simulink model "beam_mass_simulink_old"  (R2017a)
settings: Solver=FixedStepAuto  StartTime=0.0  StopTime=100  FixedStep=0.01  RelTol=1e-3
libraries: simulink_extras x2, simulink x1
settings Model: Creator=gladstonjoseph  LastModifiedBy=gladstonjoseph
settings DataIOCC: ReturnWorkspaceOutputs=on
settings DebuggingCC: UnconnectedInputMsg=none  UnconnectedOutputMsg=none  UnconnectedLineMsg=none
settings ModelReferenceCC: EnableRefExpFcnMdlSchedulingChecks=off
settings SFSimCC: SimUseLocalCustomCode=on
settings RTWCC: RTWUseLocalCustomCode=on

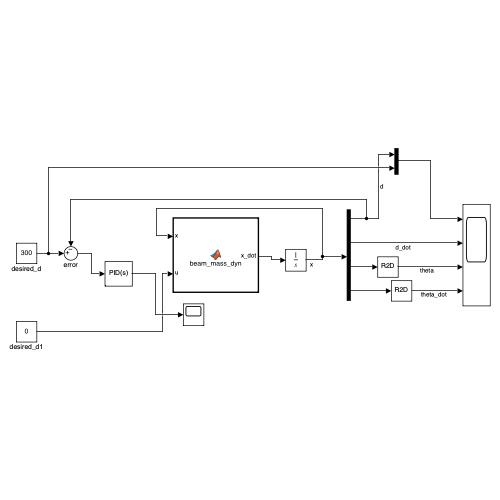
[thumbnail: Simulink's stored preview of the top-level diagram]
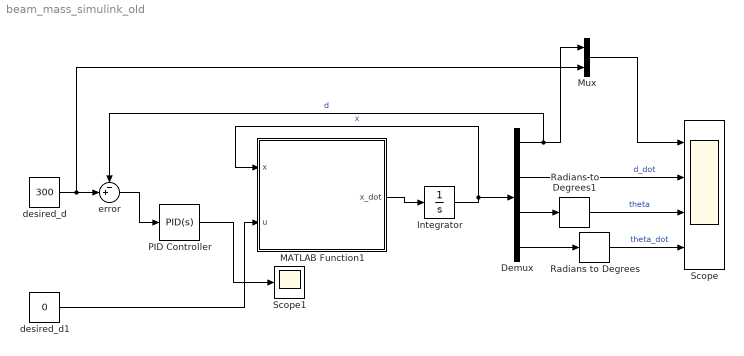
== system beam_mass_simulink_old ==
  Demux : Demux
  Integrator : Integrator  InitialCondition=[0, 0, 0.0001, 0]'
  MATLAB Function1 : MATLAB Function  TreatAsAtomicUnit=on
  Mux : Mux  Inputs=2
  PID Controller : simulink/Continuous/PID Controller  Controller=PID  Form=Parallel  TimeDomain=Continuous-time  SampleTime=-1  IntegratorMethod=Forward Euler  FilterMethod=Forward Euler  ControllerParametersSource=internal  P=0  I=20  D=0  N=100  UseFilter=on  InitialConditionSource=internal  InitialConditionForIntegrator=0  InitialConditionForFilter=0  DifferentiatorICPrevScaledInput=0  ExternalReset=none  TrackingMode=off  Kt=1  LimitOutput=off  UpperSaturationLimit=inf  LowerSaturationLimit=-inf  LinearizeAsGain=on  AntiWindupMode=none  Kb=1  POutMin=[]  POutMax=[]  IOutMin=[]  IOutMax=[]  DOutMin=[]  DOutMax=[]  NOutMin=[]  NOutMax=[]  SumOutMin=[]  SumOutMax=[]  SaturationOutMin=[]  SaturationOutMax=[]  PParamMin=[]  PParamMax=[]  IParamMin=[]  IParamMax=[]  DParamMin=[]  DParamMax=[]  NParamMin=[]  NParamMax=[]  KbParamMin=[]  KbParamMax=[]  KtParamMin=[]  KtParamMax=[]  KbOutMin=[]  KbOutMax=[]  KtOutMin=[]  KtOutMax=[]  IntegratorOutMin=[]  IntegratorOutMax=[]  FilterOutMin=[]  FilterOutMax=[]  SumI1OutMin=[]  SumI1OutMax=[]  SumI2OutMin=[]  SumI2OutMax=[]  SumI3OutMin=[]  SumI3OutMax=[]  SumDOutMin=[]  SumDOutMax=[]  DifferentiatorOutMin=[]  DifferentiatorOutMax=[]  IntegratorContinuousStateAttributes=''  IntegratorStateMustResolveToSignalObject=off  IntegratorRTWStateStorageClass=Auto  FilterContinuousStateAttributes=''  FilterStateMustResolveToSignalObject=off  FilterRTWStateStorageClass=Auto  InitialConditionSetting=State (most efficient)
  Radians to Degrees : simulink_extras/Transformations/Radians to Degrees
  Radians to Degrees1 : simulink_extras/Transformations/Radians to Degrees
  Scope : Scope  NumInputPorts=4
  Scope1 : Scope
  desired_d : Constant  Value=300
  desired_d1 : Constant  Value=0
  error : Sum  Inputs=-+|
  wires:
  MATLAB Function1/1(x_dot) -> Integrator/1
  Integrator/1 -> MATLAB Function1/1(x), Demux/1  "x"
  Demux/3 -> Radians to Degrees1/1
  Demux/1 -> Mux/1, error/1  "d"
  Demux/2 -> Scope/2  "d_dot"
  Demux/4 -> Radians to Degrees/1
  Radians to Degrees/1 -> Scope/4  "theta_dot"
  Radians to Degrees1/1 -> Scope/3  "theta"
  desired_d/1 -> Mux/2, error/2
  error/1 -> PID Controller/1
  Mux/1 -> Scope/1
  PID Controller/1 -> Scope1/1
  desired_d1/1 -> MATLAB Function1/2(u)

== matlab function beam_mass_simulink_old/MATLAB Function1 ==
  data: x input; u input; x_dot output
function x_dot = beam_mass_dyn(x, u)
    % Constants
    g = 9.81; % Gravity
    m = 5; % Mass
    J = 50; % Moment of inertia
    k = 15; % Spring constant
    c = 20; % Damping coefficient
    
    % States
    d = x(1);
    d_dot = x(2);
    theta = x(3);
    theta_dot = x(4);
    
    % Motor force
    tau = u;
    
    
    x_dot = zeros(4, 1);
    x_dot(1) = d_dot;
    x_dot(2) = -g * sin(theta);
    x_dot(3) = theta_dot;
    x_dot(4) = (tau - k * theta - c * theta_dot - m * g * d * cos(theta)) / J;
end
